simulink library "motion"  (Simulink 4.00)
undefined symbols (not defined in the file or in its folder): A6, Ac, Acd, ad, Aff, Aff0, Aff6, Ap, As, B6, Bc, Bcd, Bff, Bff0, Bff6, Bp, Bs, C6, Cc, Ccd, Cff, Cff0, Cff6, Cp, Cs, D6, Dc, dd, Ddd, Dff, Dff0, Dff6, Dp, Ds, jd, Ts, Tsettle
libraries: motion x5
(part 1 of 4)
settings Model: LastModifiedBy=plambrec

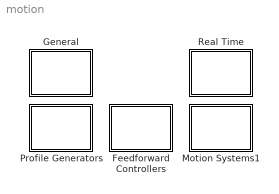
== system motion ==
  Feedforward Controllers : Subsystem
      settings: RTWFcnNameOpts=Auto  RTWFileNameOpts=Auto
      mask Display: disp('Feedforward\nControllers')
  General : Subsystem
      settings: RTWFcnNameOpts=Auto  RTWFileNameOpts=Auto
      mask Display: disp('General')
  Motion Systems1 : Subsystem
      settings: RTWFcnNameOpts=Auto  RTWFileNameOpts=Auto
      mask Display: disp('Motion\nSystems')
  Profile Generators : Subsystem
      settings: RTWFcnNameOpts=Auto  RTWFileNameOpts=Auto
      mask Display: disp('Profile\nGenerators')
  Real Time : Subsystem
      settings: RTWFcnNameOpts=Auto  RTWFileNameOpts=Auto
      mask Display: disp('Real\nTime')

== system motion/Feedforward Controllers ==
  note: Drag Template to
      | Simulink Model Window
  2nd order continuous : Subsystem  mask(Continuous Time Feedforward){m1=30, k1=20}
      mask prompts: m1 "Mass [kg]"; k1 "Actuator to ground Damping [Ns/m]"
      mask help: Continuous Time Feedforward to be used with 2nd order profile generator.
      mask init:
      | m2=0;k2=0;c=1;k12=0;
      | q3=(m1+m2)*c+k1*k2+(k1+k2)*k12;
      | q4=(k1+k2)*c;
      settings: RTWFcnNameOpts=Auto  RTWFileNameOpts=Auto
      mask Help:
      | Continuous Time Feedforward to be used with 2nd order profile generator.
      | See make2.m and look under mask.
      mask Display: disp('Cont. FF')
  2nd order discrete : Subsystem  mask(Discrete Time Feedforward){m1=20, k1=10, Ts=Ts}
      mask prompts: m1 "Actuator Mass [kg]"; k1 "Actuator to ground Damping [Ns/m]"; Ts "Sampling time [s]"
      mask help: Discrete Time Feedforward to be used with 2nd order profile generator.
      mask init:
      | m2=0;k2=0;c=1;k12=0;
      | q2=0;
      settings: RTWFcnNameOpts=Auto  RTWFileNameOpts=Auto
      mask Help:
      | Discrete Time Feedforward to be used with 2nd order profile generator.
      | See make2.m and look under mask.
      mask Display: disp('Disc. FF')
  3d order continuous : Subsystem  mask(Continuous Time Feedforward){m1=30, k1=20, q2=0}
      mask prompts: m1 "Mass [kg]"; k1 "Actuator to ground Damping [Ns/m]"; q2 "Jerk feedforward term (default 0)"
      mask help: Continuous Time Feedforward to be used with 3d order profile generator.
      mask init:
      | m2=0;k2=0;c=1;k12=0;
      | q3=(m1+m2)*c+k1*k2+(k1+k2)*k12;
      | q4=(k1+k2)*c;
      settings: RTWFcnNameOpts=Auto  RTWFileNameOpts=Auto
      mask Help:
      | Continuous Time Feedforward to be used with 3d order profile generator.
      | See make3.m and profile3.m and look under mask.
      mask Display: disp('Cont. FF')
  3d order discrete : Subsystem  mask(Discrete Time Feedforward){m1=20, k1=10, q2=0, Ts=Ts}
      mask prompts: m1 "Actuator Mass [kg]"; k1 "Actuator to ground Damping [Ns/m]"; q2 "Jerk feedforward term (default 0)"; Ts "Sampling time [s]"
      mask help: Discrete Time Feedforward to be used with 3d order profile generator.
      mask init:
      | m2=0;k2=0;c=1;k12=0;
      settings: RTWFcnNameOpts=Auto  RTWFileNameOpts=Auto
      mask Help:
      | Discrete Time Feedforward to be used with 3d order profile generator.
      | See make3.m and profile3.m and look under mask.
      mask Display: disp('Disc. FF')
  4th order  continuous x1 : Subsystem  mask(Continuous Time Feedforward){m1=20, m2=10, k1=10, k2=10, c=6e5, k12=500}
      mask prompts: m1 "Actuator Mass [kg]"; m2 "Load Mass [kg]"; k1 "Actuator to ground Damping [Ns/m]"; k2 "Load to ground Damping [Ns/m]"; c "Spring Stiffness [N/m]"; k12 "Internal Damping [Ns/m]"
      mask help: Continuous Time Feedforward to be used with 4th order profile generator.
      mask init:
      | q1=m1*m2;
      | q2=(m1+m2)*k12+m1*k2+m2*k1;
      | q3=(m1+m2)*c+k1*k2+(k1+k2)*k12;
      | q4=(k1+k2)*c;
      settings: RTWFcnNameOpts=Auto  RTWFileNameOpts=Auto
      mask Help:
      | Continuous Time Feedforward to be used with 4th order profile generator.
      | See make4.m and profile4.m and look under mask.
      mask Display: disp('Cont. FF')
  4th order  discrete x1 : Subsystem  mask(Discrete Time Feedforward){m1=20, m2=10, k1=10, k2=10, c=6e5, k12=500, Ts=Ts}
      mask prompts: m1 "Actuator Mass [kg]"; m2 "Load Mass [kg]"; k1 "Actuator to ground Damping [Ns/m]"; k2 "Load to ground Damping [Ns/m]"; c "Spring Stiffness [N/m]"; k12 "Internal Damping [Ns/m]"; Ts "Sampling time [s]"
      mask help: Discrete Time Feedforward to be used with 4th order profile generator.
      settings: RTWFcnNameOpts=Auto  RTWFileNameOpts=Auto
      mask Help:
      | Discrete Time Feedforward to be used with 4th order profile generator.
      | See make4.m and profile4.m and look under mask.
      mask Display: disp('Disc. FF')
  4th order continuous : Subsystem  mask(Continuous Time Feedforward){m1=20, m2=10, k1=10, k2=10, c=6e5, k12=500}
      mask prompts: m1 "Actuator Mass [kg]"; m2 "Load Mass [kg]"; k1 "Actuator to ground Damping [Ns/m]"; k2 "Load to ground Damping [Ns/m]"; c "Spring Stiffness [N/m]"; k12 "Internal Damping [Ns/m]"
      mask help: Continuous Time Feedforward to be used with 4th order profile generator.
      mask init:
      | q1=m1*m2;
      | q2=(m1+m2)*k12+m1*k2+m2*k1;
      | q3=(m1+m2)*c+k1*k2+(k1+k2)*k12;
      | q4=(k1+k2)*c;
      settings: RTWFcnNameOpts=Auto  RTWFileNameOpts=Auto
      mask Help:
      | Continuous Time Feedforward to be used with 4th order profile generator.
      | See make4.m and profile4.m and look under mask.
      mask Display: disp('Cont. FF')
  4th order digital : Subsystem  mask(Digital Feedforward){m1=20, m2=10, k1=10, k2=10, c=6e5, k12=500, Ts=Ts, r=10*eps}
      mask prompts: m1 "Actuator Mass [kg]"; m2 "Load Mass [kg]"; k1 "Actuator to ground Damping [Ns/m]"; k2 "Load to ground Damping [Ns/m]"; c "Spring Stiffness [N/m]"; k12 "Internal Damping [Ns/m]"; Ts "Sampling time [s]"; r "Resolution of position [m] (default: 10*eps)"
      mask help: Digital Feedforward to be used with 4th order profile generator.
      settings: RTWFcnNameOpts=Auto  RTWFileNameOpts=Auto
      mask Help:
      | Digital Feedforward to be used with 4th order profile generator.
      | See make4.m and profile4.m and look under mask.
      mask Display: disp('Dig. FF')
  4th order discrete : Subsystem  mask(Discrete Time Feedforward){m1=20, m2=10, k1=10, k2=10, c=6e5, k12=500, Ts=Ts}
      mask prompts: m1 "Actuator Mass [kg]"; m2 "Load Mass [kg]"; k1 "Actuator to ground Damping [Ns/m]"; k2 "Load to ground Damping [Ns/m]"; c "Spring Stiffness [N/m]"; k12 "Internal Damping [Ns/m]"; Ts "Sampling time [s]"
      mask help: Discrete Time Feedforward to be used with 4th order profile generator.
      settings: RTWFcnNameOpts=Auto  RTWFileNameOpts=Auto
      mask Help:
      | Discrete Time Feedforward to be used with 4th order profile generator.
      | See make4.m and profile4.m and look under mask.
      mask Display: disp('Disc. FF')
  Feedforward : Subsystem  BlockChoice=4th order continuous
      settings: TemplateBlock=self  MemberBlocks=2nd order continuous,2nd order discrete,3d order continuous,3d order discrete,4th order continuous,4th order digital,4th order discrete  RTWFcnNameOpts=Auto  RTWFileNameOpts=Auto

== system motion/General ==
  note: used to specify parameters
      | for blocks below
  2nd order plant : StateSpace  A=As  B=Bs  C=Cs  D=Ds  X0=0  Realization=auto  AbsoluteTolerance=auto
  4th order Digital Feedforward : Subsystem  mask(4th Order Digital Feedforward ){t0=.3, x=1, v=1, a=5, j=50, d=1000, Ts=1e-3, r=10*eps, s=15, m1=20, m2=10, k1=10, k2=10, c=6e5, k12=500}
      mask prompts: t0 "Starting time:  t0 [s]"; x "Displacement:  x [m]"; v "Bound on velocity:  vmax [m/s]"; a "Bound on acceleration:  amax [m/s2]"; j "Bound on jerk: jmax [m/s3]"; d "Bound on derivative of jerk:  dmax [m/s4]"; Ts "Sampling time (0 for continuous):  Ts [s]"; r "Resolution of position [m] (default: 10*eps)"; s "Number of decimals for digitized d (default: 15)"; m1 "Actuator Mass [kg]"; m2 "Load Mass [kg]"; k1 "Actuator to ground Damping [Ns/m]"; k2 "Load to ground Damping [Ns/m]"; c "Spring Stiffness [N/m]"; k12 "Internal Damping [Ns/m]"
      mask help: Implements a 4th order trajectory planner and feedforward calculation.
      mask init:
      | if length(r)==0 | length(s)==0
      | 	r=10*eps;
      | 	s=15;
      | end
      | [t,dd]=make4(abs(x),v,a,j,d,Ts,r,s);
      | t01=t0-10*eps;
      | if Ts==0
      |    [dj1,tx1,d1,j1,a1,v1,p1,tt1]=profile4(t,dd(1),.001,0);
      | else
      |    [dj1,tx1,d1,j1,a1,v1,p1,tt1]=profile4(t,dd(1),Ts/10,0);
      | end
      settings: RTWFcnNameOpts=Auto  RTWFileNameOpts=Auto
      mask Help: Look under mask
      mask Display:
      | plot([0 dj1(1,:)+t0],[0 dj1(2,:)])
      | text(0.9*(max(dj1(1,:))+t0),0,'F\nx')
  4th order plant : StateSpace  A=Ap  B=Bp  C=Cp  D=Dp  X0=0  Realization=auto  AbsoluteTolerance=auto
  6th order plant : StateSpace  A=A6  B=B6  C=C6  D=D6  X0=0  Realization=auto  AbsoluteTolerance=auto
  Controller : StateSpace  A=Ac  B=Bc  C=Cc  D=Dc  X0=0  Realization=auto  AbsoluteTolerance=auto
  Discrete controller : DiscreteStateSpace  A=Acd  B=Bcd*1.4  C=Ccd  D=Ddd  X0=0  SampleTime=Ts  Realization=auto
  FF: 4th order k12=0 : StateSpace  A=Aff0  B=Bff0  C=Cff0  D=Dff0  X0=0  Realization=auto  AbsoluteTolerance=auto
  FF: 6th order tuning : StateSpace  A=Aff6  B=Bff6  C=Cff6  D=Dff6  X0=0  Realization=auto  AbsoluteTolerance=auto
  FF: Ideal 4th order : StateSpace  A=Aff  B=Bff  C=Cff  D=Dff  X0=0  Realization=auto  AbsoluteTolerance=auto
  open example : Subsystem
      settings: OpenFcn=motion_example1  RTWFcnNameOpts=Auto  RTWFileNameOpts=Auto
      mask Type: Model Opener
      mask Description: Opens Simulink model
      mask Display: disp('EXAMPLE 1\ndoubleclick to open')
  open example1 : Subsystem
      settings: RTWFcnNameOpts=Auto  RTWFileNameOpts=Auto
      settings: OpenFcn=|
      | makeplant
      | motion_example3
      mask Type: Model Opener
      mask Description: Opens Simulink model
      mask Display: disp('EXAMPLE 3\ndoubleclick to open')
  open example2 : Subsystem
      settings: RTWFcnNameOpts=Auto  RTWFileNameOpts=Auto
      settings: OpenFcn=|
      | makeplant
      | motion_example2
      mask Type: Model Opener
      mask Description: Opens Simulink model
      mask Display: disp('EXAMPLE 2\ndoubleclick to open')
  run makeplant : Subsystem
      settings: OpenFcn=makeplant  MoveFcn=edit makeplant  RTWFcnNameOpts=Auto  RTWFileNameOpts=Auto
      mask Type: Script Runner
      mask Description: Run Matlab .M script
      mask Help:
      | This is a convenient block to edit and run a Matlab .M scriptfile from the Simulink environment.
      | Typically such a script is used to define simulation and system parameters.
      | 
      | As an example the scriptfile MAKEPLANT.m is supplied: you may edit this file or use your own.
      | 
      | Double clicking this block will run the script, moving it will start the Matlab editor.
      | 
      | A different script file name can be specified by editing the Callback functions OpenFcn and MoveFcn
      | (see Block Properties)
      mask Display: disp('MAKEPLANT\ndoubleclick to run\nmove to edit')

== system motion/Motion Systems1 ==
  note: Drag Template to
      | Simulink Model Window
  2nd order : StateSpace  A=As  B=Bs  C=Cs  D=Ds  X0=0  Realization=auto  AbsoluteTolerance=auto
  4th order : StateSpace  A=Ap  B=Bp  C=Cp  D=Dp  X0=0  Realization=auto  AbsoluteTolerance=auto
  6th order : StateSpace  A=A6  B=B6  C=C6  D=D6  X0=0  Realization=auto  AbsoluteTolerance=auto
  Motion System : Subsystem  BlockChoice=2nd order
      settings: TemplateBlock=self  MemberBlocks=2nd order,4th order,6th order,Parametrized 4th order  RTWFcnNameOpts=Auto  RTWFileNameOpts=Auto
  Parametrized 4th order : Subsystem  mask(Parametrized 4th order motion system model){m1=20, m2=10, k1=100, k2=100, c=6e5, k12=500}
      mask prompts: m1 "Actuator Mass [kg]"; m2 "Load Mass [kg]"; k1 "Actuator to ground Damping [Ns/m]"; k2 "Load to ground Damping [Ns/m]"; c "Spring Stiffness [N/m]"; k12 "Internal Damping [Ns/m]"
      mask help: Parametrized 4th order motion system model
      mask init:
      | Ap = [   0         1         0         0             % x1
      |        -c/m1  -(k1+k12)/m1  c/m1     k12/m1          % x1dot
      |          0         0         0         1             % x2
      |         c/m2     k12/m2    -c/m2  -(k2+k12)/m2 ];    % x2dot
      | Bp = [   0
      |         1/m1     
      |          0
      |          0   ];
      | Cp = [   0         0        1         0     ];      % x2
      | Dp=0;
      settings: RTWFcnNameOpts=Auto  RTWFileNameOpts=Auto
      mask Help: Parametrized 4th order motion system model
      mask Display: disp('4th order')

== system motion/Profile Generators ==
  note: Drag Template to
      | Simulink Model Window
  Acceleration : Subsystem  mask(2nd Order Profile Generator){t0=.3, x=1, v=1, a=5, Ts=0}
      mask prompts: t0 "Starting time:  t0 [s]"; x "Displacement:  x [m]"; v "Bound on velocity:  vmax [m/s]"; a "Bound on acceleration:  amax [m/s2]"; Ts "Sampling time (0 for continuous):  Ts [s]"
      mask help: 2nd Order Profile Generator
      mask init:
      | [t,ad,aa,tx,a,v,p,tt] = make2(abs(x),v,a,Ts,0);
      | t0=t0-10*eps;
      settings: RTWFcnNameOpts=Auto  RTWFileNameOpts=Auto
      mask Help: See make2.m and look under mask
      mask Display:
      | plot([0 aa(1,:)+t0],[0 aa(2,:)])
      | text(0.8*(max(aa(1,:))+t0),0,'a\n')
  Derivative of Jerk : Subsystem  AncestorBlock=library/Derivative of jerk profile generator  mask(4th Order Profile Generator){t0=.3, x=1, v=1, a=5, j=50, d=1000, Ts=0}
      mask prompts: t0 "Starting time:  t0 [s]"; x "Displacement:  x [m]"; v "Bound on velocity:  vmax [m/s]"; a "Bound on acceleration:  amax [m/s2]"; j "Bound on jerk: jmax [m/s3]"; d "Bound on derivative of jerk:  dmax [m/s4]"; Ts "Sampling time (0 for continuous):  Ts [s]"
      mask help: 4th Order Profile Generator
      mask init:
      | [t,dd]=make4(abs(x),v,a,j,d,Ts);
      | t0=t0-10*eps;
      | [dj,tx,d,j,a,v,p,tt]=profile4(t,dd(1),0,0);
      settings: RTWFcnNameOpts=Auto  RTWFileNameOpts=Auto
      mask Help: See make4.m and profile4.m and look under mask
      mask Display:
      | plot([0 dj(1,:)+t0],[0 dj(2,:)])
      | text(0.8*(max(dj(1,:))+t0),0,'d\n')
  Jerk : Subsystem  mask(3d Order Profile Generator){t0=.3, x=1, v=1, a=5, j=50, Ts=0}
      mask prompts: t0 "Starting time:  t0 [s]"; x "Displacement:  x [m]"; v "Bound on velocity:  vmax [m/s]"; a "Bound on acceleration:  amax [m/s2]"; j "Bound on jerk: jmax [m/s3]"; Ts "Sampling time (0 for continuous):  Ts [s]"
      mask help: 3d Order Profile Generator
      mask init:
      | [t,jd]=make3(abs(x),v,a,j,Ts);
      | t0=t0-10*eps;
      | [jj,tx,j,a,v,p,tt]=profile3(t,jd(1),0,0);
      settings: RTWFcnNameOpts=Auto  RTWFileNameOpts=Auto
      mask Help: See make3.m and profile3.m and look under mask
      mask Display:
      | plot([0 jj(1,:)+t0],[0 jj(2,:)])
      | text(0.85*(max(jj(1,:))+t0),0,'j\n')
  Profile Generator : Subsystem  BlockChoice=Acceleration
      settings: TemplateBlock=self  MemberBlocks=Acceleration,Derivative of Jerk,Jerk,dJerk with error correction  RTWFcnNameOpts=Auto  RTWFileNameOpts=Auto
  dJerk with error correction : Subsystem  mask(4th Order Profile Generator with quantization error correction){t0=.3, x=1, v=1, a=5, j=50, d=1000, Ts=0, r=10*eps, s=15}
      mask prompts: t0 "Starting time:  t0 [s]"; x "Displacement:  x [m]"; v "Bound on velocity:  vmax [m/s]"; a "Bound on acceleration:  amax [m/s2]"; j "Bound on jerk: jmax [m/s3]"; d "Bound on derivative of jerk:  dmax [m/s4]"; Ts "Sampling time (0 for continuous):  Ts [s]"; r "Resolution of position [m] (default: 10*eps)"; s "Number of decimals for digitized d (default: 15)"
      mask help: 4th Order Profile Generator with quantization error correction
      mask init:
      | if length(r)==0 | length(s)==0
      | 	r=10*eps;
      | 	s=15;
      | end
      | [t,dd]=make4(abs(x),v,a,j,d,Ts,r,s);
      | t0=t0-10*eps;
      | [dj,tx,d,j,a,v,p,tt]=profile4(t,dd(1),0,0);
      settings: RTWFcnNameOpts=Auto  RTWFileNameOpts=Auto
      mask Help: See make4.m and profile4.m and look under mask
      mask Display:
      | plot([0 dj(1,:)+t0],[0 dj(2,:)])
      | text(0.8*(max(dj(1,:))+t0),0,'d\n')

== system motion/Real Time ==
  1 : Constant  Value=1
  2 : Constant  Value=0
  Demux : Demux  Outputs=[1 1 5]  BusSelectionMode=off
  Demux1 : Demux  Outputs=[1 1 5]  BusSelectionMode=off
  Generate Feedforward : Subsystem  mask{m1=20, m2=10, k1=10, k2=10, c=6e5, k12=500, Ts=Ts, S1=1, S2=1}
      mask prompts: m1 "Actuator Mass [kg]"; m2 "Load Mass [kg]"; k1 "Actuator Damping [Ns/m]"; k2 "Load Damping [Ns/m]"; c "Stiffness [N/m]"; k12 "Internal Damping [Ns/m]"; Ts "Sample Time [s]"; S1 "Select: 4th order(1) or rigid body(0)"; S2 "Select: actuator(1) or load(0) pos mmnt"
      settings: RTWFcnNameOpts=Auto  RTWFileNameOpts=Auto
  Generate Feedforward with reset : Subsystem  mask{m1=20, m2=10, k1=10, k2=10, c=6e5, k12=500, Ts=Ts, S1=1, S2=1}
      mask prompts: m1 "Actuator Mass [kg]"; m2 "Load Mass [kg]"; k1 "Actuator Damping [Ns/m]"; k2 "Load Damping [Ns/m]"; c "Stiffness [N/m]"; k12 "Internal Damping [Ns/m]"; Ts "Sample Time [s]"; S1 "Select: 4th order(1) or rigid body(0)"; S2 "Select: actuator(1) or load(0) pos mmnt"
      settings: RTWFcnNameOpts=Auto  RTWFileNameOpts=Auto
  Generate Profile : Subsystem  mask{Ts=Ts, Tset=Tsettle, Sdir=1}
      mask prompts: Ts "Sample time [s]"; Tset "Settling time [s]"; Sdir "Switch direction when enabled: 1/0"
      settings: RTWFcnNameOpts=Auto  RTWFileNameOpts=Auto
  Generate Profile with reset : Subsystem  mask{Ts=Ts, Tset=Tsettle, Sdir=1}
      mask prompts: Ts "Sample time [s]"; Tset "Settling time [s]"; Sdir "Switch direction when enabled: 1/0"
      settings: RTWFcnNameOpts=Auto  RTWFileNameOpts=Auto
  Memory1 : Memory  X0=0  InheritSampleTime=on
  Memory2 : Memory  X0=0  InheritSampleTime=on
  Plan Trajectory : Subsystem  TreatAsAtomicUnit=on
      settings: RTWFcnNameOpts=Auto  RTWFileNameOpts=Auto
  Plan Trajectory (with displays) : Subsystem  TreatAsAtomicUnit=on
      settings: RTWFcnNameOpts=Auto  RTWFileNameOpts=Auto
  Terminator1 : Terminator
  Terminator7 : Terminator
  "X-Y planner " : Subsystem  mask{Ts=1/4000, Tsettle=1, X=[ 0 0 ; 0.2 0.2 ; 0.2 -0.2 ; -0.2 -0.2 ; -0.2 0.2 ]}
      mask prompts: Ts "Sampling time [s]"; Tsettle "Settling time (after each move) [s]"; X "Waypoints [ [x1 y1] ; [x2 y2] ; .....]"
      settings: RTWFcnNameOpts=Auto  RTWFileNameOpts=Auto
  open example : Subsystem
      settings: OpenFcn=ref4_rt  RTWFcnNameOpts=Auto  RTWFileNameOpts=Auto
      mask Type: Model Opener
      mask Description: Opens Simulink model
      mask Display: disp('EXAMPLE\ndoubleclick to open')
  open example1 : Subsystem
      settings: OpenFcn=ref4_xy  RTWFcnNameOpts=Auto  RTWFileNameOpts=Auto
      mask Type: Model Opener
      mask Description: Opens Simulink model
      mask Display: disp('EXAMPLE\ndoubleclick to open')
  wires:
  Generate Profile/1(djerk) -> Generate Feedforward/1(djerk)
  Generate Profile with reset/2(reset) -> Generate Feedforward with reset/2(reset)
  Generate Profile with reset/1(djerk) -> Generate Feedforward with reset/1(djerk)
  Generate Profile/2(start) -> Plan Trajectory/Trigger
  Memory2/1 -> Generate Profile/1(t,d)
  Plan Trajectory/1(t,d) -> Memory2/1
  Generate Profile with reset/3(start) -> Plan Trajectory (with displays)/Trigger
  Memory1/1 -> Generate Profile with reset/1(t,d)
  Plan Trajectory (with displays)/1(t,d) -> Memory1/1
  Demux/2 -> [Xref]
  Demux/3 -> Terminator7/1
  Demux/1 -> [FffX]
  "X-Y planner "/1(X) -> Demux/1
  Demux1/2 -> [Yref]
  Demux1/3 -> Terminator1/1
  Demux1/1 -> [FffY]
  "X-Y planner "/2(Y) -> Demux1/1
  1/1 -> "X-Y planner "/1("Cont ")
  2/1 -> "X-Y planner "/2(Trig)

== system motion/Feedforward Controllers/2nd order continuous ==
  note: Rigid Body Feedforward
  note: a
  In1 : Inport  Port=1
  Constant : Constant  Value=0
  Constant1 : Constant  Value=0
  Mux : Mux  Inputs=7
  Position : Integrator  ExternalReset=none  InitialConditionSource=internal  InitialCondition=0  LimitOutput=off  UpperSaturationLimit=inf  LowerSaturationLimit=-inf  ShowSaturationPort=off  ShowStatePort=off  AbsoluteTolerance=auto
  Sum2 : Sum  Orientation=down  Inputs=++|  SaturateOnIntegerOverflow=on
  Velocity : Integrator  ExternalReset=none  InitialConditionSource=internal  InitialCondition=0  LimitOutput=off  UpperSaturationLimit=inf  LowerSaturationLimit=-inf  ShowSaturationPort=off  ShowStatePort=off  AbsoluteTolerance=auto
  filter : TransferFcn  Orientation=down  Numerator=[1]  Denominator=[c]  Realization=auto  AbsoluteTolerance=auto
  m : Gain  Gain=q3  Multiplication=Element-wise(K.*u)  SaturateOnIntegerOverflow=on
  m1 : Gain  Gain=q4  Multiplication=Element-wise(K.*u)  SaturateOnIntegerOverflow=on
  rigid body : Subsystem
      settings: RTWFcnNameOpts=Auto  RTWFileNameOpts=Auto
      mask Display: disp('')
  Out1 : Outport  Port=1
  wires:
  Mux/1 -> Out1/1
  filter/1 -> Mux/1  "feedforward force"
  m/1 -> Sum2/2
  m1/1 -> Sum2/1
  Sum2/1 -> filter/1
  Position/1 -> Mux/2, [p]  "reference"
  Velocity/1 -> Position/1, m1/1, [v]
  In1/1 -> Velocity/1, m/1, [a]
  [p] -> Mux/7  "position"
  Constant/1 -> Mux/3  "derivative of jerk"
  Constant1/1 -> Mux/4  "jerk"
  [a] -> Mux/5  "acceleration"
  [v] -> Mux/6  "velocity"

== system motion/Feedforward Controllers/2nd order discrete ==
  In1 : Inport  Port=1
  (k1+k2)*c : Gain  Gain=(k1+k2)*c  Multiplication=Element-wise(K.*u)  SaturateOnIntegerOverflow=on
  (m1+m2)*c+k1*k2+(k1+k2)*k12 : Gain  Gain=(m1+m2)*c+k1*k2+(k1+k2)*k12  Multiplication=Element-wise(K.*u)  SaturateOnIntegerOverflow=on
  1/c : Gain  Gain=1/c  Multiplication=Element-wise(K.*u)  SaturateOnIntegerOverflow=on
  Constant{,1..3} (4 alike) : Constant  Value=0
  Discrete variable delay : Subsystem  mask{Ts=Ts, alpha=.5}
      mask prompts: Ts "Sample time"; alpha "Delay factor (between 0 and 1)"
      settings: RTWFcnNameOpts=Auto  RTWFileNameOpts=Auto
      mask Display: disp(sprintf('%3.1f*Ts',alpha))
  Discrete variable delay1 : Subsystem  mask{Ts=Ts, alpha=.5}
      mask prompts: Ts "Sample time"; alpha "Delay factor (between 0 and 1)"
      settings: RTWFcnNameOpts=Auto  RTWFileNameOpts=Auto
      mask Display: disp(sprintf('%3.1f*Ts',alpha))
  Discrete variable delay2 : Subsystem  mask{Ts=Ts, alpha=.5}
      mask prompts: Ts "Sample time"; alpha "Delay factor (between 0 and 1)"
      settings: RTWFcnNameOpts=Auto  RTWFileNameOpts=Auto
      mask Display: disp(sprintf('%3.1f*Ts',alpha))
  Mux1 : Mux  Inputs=3
  Mux2 : Mux  Inputs=5
  Sum1 : Sum  Inputs=++++  SaturateOnIntegerOverflow=on
  Unit Delay{1..3,5} (4 alike) : UnitDelay  X0=0  SampleTime=Ts
  ZOH1 : ZeroOrderHold  SampleTime=Ts
  m1*m2 : Gain  Gain=m1*m2  Multiplication=Element-wise(K.*u)  SaturateOnIntegerOverflow=on
  position : DiscreteIntegrator  IntegratorMethod=ForwardEuler  ExternalReset=none  InitialConditionSource=internal  InitialCondition=0  LimitOutput=off  UpperSaturationLimit=inf  LowerSaturationLimit=-inf  ShowSaturationPort=off  ShowStatePort=off  SampleTime=Ts
  q2 : Gain  Gain=q2  Multiplication=Element-wise(K.*u)  SaturateOnIntegerOverflow=on
  velocity : DiscreteIntegrator  IntegratorMethod=ForwardEuler  ExternalReset=none  InitialConditionSource=internal  InitialCondition=0  LimitOutput=off  UpperSaturationLimit=inf  LowerSaturationLimit=-inf  ShowSaturationPort=off  ShowStatePort=off  SampleTime=Ts
  Out1 : Outport  Port=1
  wires:
  [mon] -> Mux1/3
  [ref] -> Mux1/2
  [force] -> Mux1/1
  Mux1/1 -> Out1/1
  Mux2/1 -> [mon]
  velocity/1 -> position/1, [v]
  ZOH1/1 -> velocity/1, [a]  "derivative of jerk"
  position/1 -> [p]
  [p] -> Mux2/5  "position"
  Constant/1 -> Mux2/1  "derivative of jerk"
  Constant3/1 -> Mux2/2  "jerk"
  [a] -> Mux2/3  "acceleration"
  [v] -> Mux2/4  "velocity"
  Constant1/1 -> Unit Delay5/1
  Constant2/1 -> Unit Delay2/1
  [a] -> Unit Delay3/1
  [v] -> Discrete variable delay1/1(In1)
  (m1+m2)*c+k1*k2+(k1+k2)*k12/1 -> Sum1/3
  (k1+k2)*c/1 -> Sum1/4
  Sum1/1 -> 1/c/1
  [p] -> Discrete variable delay/1(In1)
  Discrete variable delay/1(Out1) -> [ref]
  Unit Delay5/1 -> Unit Delay1/1
  Unit Delay1/1 -> m1*m2/1
  Unit Delay2/1 -> Discrete variable delay2/1(In1)
  Unit Delay3/1 -> (m1+m2)*c+k1*k2+(k1+k2)*k12/1
  Discrete variable delay1/1(Out1) -> (k1+k2)*c/1
  Discrete variable delay2/1(Out1) -> q2/1
  1/c/1 -> [force]
  q2/1 -> Sum1/2
  m1*m2/1 -> Sum1/1
  In1/1 -> ZOH1/1

== system motion/Feedforward Controllers/3d order continuous ==
  note: j
  note: Rigid Body Feedforward
  In1 : Inport  Port=1
  Acceleration : Integrator  ExternalReset=none  InitialConditionSource=internal  InitialCondition=0  LimitOutput=off  UpperSaturationLimit=inf  LowerSaturationLimit=-inf  ShowSaturationPort=off  ShowStatePort=off  AbsoluteTolerance=auto
  Constant : Constant  Value=0
  Mux : Mux  Inputs=7
  Position : Integrator  ExternalReset=none  InitialConditionSource=internal  InitialCondition=0  LimitOutput=off  UpperSaturationLimit=inf  LowerSaturationLimit=-inf  ShowSaturationPort=off  ShowStatePort=off  AbsoluteTolerance=auto
  Sum2 : Sum  Orientation=down  Inputs=++|  SaturateOnIntegerOverflow=on
  Sum5 : Sum  Orientation=down  Inputs=++|  SaturateOnIntegerOverflow=on
  Velocity : Integrator  ExternalReset=none  InitialConditionSource=internal  InitialCondition=0  LimitOutput=off  UpperSaturationLimit=inf  LowerSaturationLimit=-inf  ShowSaturationPort=off  ShowStatePort=off  AbsoluteTolerance=auto
  filter : TransferFcn  Orientation=down  Numerator=[1]  Denominator=[c]  Realization=auto  AbsoluteTolerance=auto
  m : Gain  Gain=q3  Multiplication=Element-wise(K.*u)  SaturateOnIntegerOverflow=on
  m1 : Gain  Gain=q4  Multiplication=Element-wise(K.*u)  SaturateOnIntegerOverflow=on
  m2 : Gain  Gain=q2  Multiplication=Element-wise(K.*u)  SaturateOnIntegerOverflow=on
  rigid body : Subsystem
      settings: RTWFcnNameOpts=Auto  RTWFileNameOpts=Auto
      mask Display: disp('')
  Out1 : Outport  Port=1
  wires:
  [v] -> Mux/6  "velocity"
  [a] -> Mux/5  "acceleration"
  [j] -> Mux/4  "jerk"
  Constant/1 -> Mux/3  "derivative of jerk"
  [p] -> Mux/7  "position"
  In1/1 -> [j], m2/1, Acceleration/1
  Velocity/1 -> [v], m1/1, Position/1
  Position/1 -> [p], Mux/2  "reference"
  Sum2/1 -> filter/1
  m1/1 -> Sum2/1
  Acceleration/1 -> [a], m/1, Velocity/1
  m/1 -> Sum5/1
  Sum5/1 -> Sum2/2
  m2/1 -> Sum5/2
  filter/1 -> Mux/1  "feedforward force"
  Mux/1 -> Out1/1

== system motion/Feedforward Controllers/3d order discrete ==
  In1 : Inport  Port=1
  (k1+k2)*c : Gain  Gain=(k1+k2)*c  Multiplication=Element-wise(K.*u)  SaturateOnIntegerOverflow=on
  (m1+m2)*c+k1*k2+(k1+k2)*k12 : Gain  Gain=(m1+m2)*c+k1*k2+(k1+k2)*k12  Multiplication=Element-wise(K.*u)  SaturateOnIntegerOverflow=on
  1/c : Gain  Gain=1/c  Multiplication=Element-wise(K.*u)  SaturateOnIntegerOverflow=on
  Constant : Constant  Value=0
  Constant1 : Constant  Value=0
  Discrete variable delay : Subsystem  mask{Ts=Ts, alpha=.5}
      mask prompts: Ts "Sample time"; alpha "Delay factor (between 0 and 1)"
      settings: RTWFcnNameOpts=Auto  RTWFileNameOpts=Auto
      mask Display: disp(sprintf('%3.1f*Ts',alpha))
  Discrete variable delay1 : Subsystem  mask{Ts=Ts, alpha=.5}
      mask prompts: Ts "Sample time"; alpha "Delay factor (between 0 and 1)"
      settings: RTWFcnNameOpts=Auto  RTWFileNameOpts=Auto
      mask Display: disp(sprintf('%3.1f*Ts',alpha))
  Discrete variable delay2 : Subsystem  mask{Ts=Ts, alpha=.5}
      mask prompts: Ts "Sample time"; alpha "Delay factor (between 0 and 1)"
      settings: RTWFcnNameOpts=Auto  RTWFileNameOpts=Auto
      mask Display: disp(sprintf('%3.1f*Ts',alpha))
  Mux1 : Mux  Inputs=3
  Mux2 : Mux  Inputs=5
  Sum1 : Sum  Inputs=++++  SaturateOnIntegerOverflow=on
  Unit Delay{1..3,5} (4 alike) : UnitDelay  X0=0  SampleTime=Ts
  ZOH1 : ZeroOrderHold  SampleTime=Ts
  acceleration : DiscreteIntegrator  IntegratorMethod=ForwardEuler  ExternalReset=none  InitialConditionSource=internal  InitialCondition=0  LimitOutput=off  UpperSaturationLimit=inf  LowerSaturationLimit=-inf  ShowSaturationPort=off  ShowStatePort=off  SampleTime=Ts
  m1*m2 : Gain  Gain=m1*m2  Multiplication=Element-wise(K.*u)  SaturateOnIntegerOverflow=on
  position : DiscreteIntegrator  IntegratorMethod=ForwardEuler  ExternalReset=none  InitialConditionSource=internal  InitialCondition=0  LimitOutput=off  UpperSaturationLimit=inf  LowerSaturationLimit=-inf  ShowSaturationPort=off  ShowStatePort=off  SampleTime=Ts
  q2 : Gain  Gain=q2  Multiplication=Element-wise(K.*u)  SaturateOnIntegerOverflow=on
  velocity : DiscreteIntegrator  IntegratorMethod=ForwardEuler  ExternalReset=none  InitialConditionSource=internal  InitialCondition=0  LimitOutput=off  UpperSaturationLimit=inf  LowerSaturationLimit=-inf  ShowSaturationPort=off  ShowStatePort=off  SampleTime=Ts
  Out1 : Outport  Port=1
  wires:
  In1/1 -> ZOH1/1
  m1*m2/1 -> Sum1/1
  q2/1 -> Sum1/2
  1/c/1 -> [force]
  Discrete variable delay2/1(Out1) -> q2/1
  Discrete variable delay1/1(Out1) -> (k1+k2)*c/1
  Unit Delay3/1 -> (m1+m2)*c+k1*k2+(k1+k2)*k12/1
  Unit Delay2/1 -> Discrete variable delay2/1(In1)
  Unit Delay1/1 -> m1*m2/1
  Unit Delay5/1 -> Unit Delay1/1
  Discrete variable delay/1(Out1) -> [ref]
  [p] -> Discrete variable delay/1(In1)
  Sum1/1 -> 1/c/1
  (k1+k2)*c/1 -> Sum1/4
  (m1+m2)*c+k1*k2+(k1+k2)*k12/1 -> Sum1/3
  [v] -> Discrete variable delay1/1(In1)
  [a] -> Unit Delay3/1
  [j] -> Unit Delay2/1
  Constant1/1 -> Unit Delay5/1
  [v] -> Mux2/4  "velocity"
  [a] -> Mux2/3  "acceleration"
  [j] -> Mux2/2  "jerk"
  Constant/1 -> Mux2/1  "derivative of jerk"
  [p] -> Mux2/5  "position"
  position/1 -> [p]
  ZOH1/1 -> [j], acceleration/1  "derivative of jerk"
  velocity/1 -> [v], position/1
  acceleration/1 -> [a], velocity/1
  Mux2/1 -> [mon]
  Mux1/1 -> Out1/1
  [force] -> Mux1/1
  [ref] -> Mux1/2
  [mon] -> Mux1/3

== system motion/Feedforward Controllers/4th order  continuous x1 ==
  note: d
  note: Rigid Body Feedforward
  In1 : Inport  Port=1
  Acceleration : Integrator  ExternalReset=none  InitialConditionSource=internal  InitialCondition=0  LimitOutput=off  UpperSaturationLimit=inf  LowerSaturationLimit=-inf  ShowSaturationPort=off  ShowStatePort=off  AbsoluteTolerance=auto
  Jerk : Integrator  ExternalReset=none  InitialConditionSource=internal  InitialCondition=0  LimitOutput=off  UpperSaturationLimit=inf  LowerSaturationLimit=-inf  ShowSaturationPort=off  ShowStatePort=off  AbsoluteTolerance=auto
  Mux : Mux  Inputs=7
  Position : Integrator  ExternalReset=none  InitialConditionSource=internal  InitialCondition=0  LimitOutput=off  UpperSaturationLimit=inf  LowerSaturationLimit=-inf  ShowSaturationPort=off  ShowStatePort=off  AbsoluteTolerance=auto
  Sum1 : Sum  Inputs=+++  SaturateOnIntegerOverflow=on
  Sum2 : Sum  Orientation=down  Inputs=++|  SaturateOnIntegerOverflow=on
  Sum3 : Sum  Orientation=down  Inputs=++|  SaturateOnIntegerOverflow=on
  Sum5 : Sum  Orientation=down  Inputs=++|  SaturateOnIntegerOverflow=on
  Velocity : Integrator  ExternalReset=none  InitialConditionSource=internal  InitialCondition=0  LimitOutput=off  UpperSaturationLimit=inf  LowerSaturationLimit=-inf  ShowSaturationPort=off  ShowStatePort=off  AbsoluteTolerance=auto
  filter : TransferFcn  Orientation=down  Numerator=[1]  Denominator=[ k12 c]  Realization=auto  AbsoluteTolerance=auto
  filter1 : TransferFcn  Numerator=[1]  Denominator=[ k12 c]  Realization=auto  AbsoluteTolerance=auto
  m : Gain  Gain=q3  Multiplication=Element-wise(K.*u)  SaturateOnIntegerOverflow=on
  m1 : Gain  Gain=q4  Multiplication=Element-wise(K.*u)  SaturateOnIntegerOverflow=on
  m2 : Gain  Gain=q2  Multiplication=Element-wise(K.*u)  SaturateOnIntegerOverflow=on
  m3 : Gain  Gain=q1  Multiplication=Element-wise(K.*u)  SaturateOnIntegerOverflow=on
  m4 : Gain  Gain=k2+k12  Multiplication=Element-wise(K.*u)  SaturateOnIntegerOverflow=on
  m5 : Gain  Gain=m2  Multiplication=Element-wise(K.*u)  SaturateOnIntegerOverflow=on
  m6 : Gain  Gain=c  Multiplication=Element-wise(K.*u)  SaturateOnIntegerOverflow=on
  rigid body : Subsystem
      settings: RTWFcnNameOpts=Auto  RTWFileNameOpts=Auto
      mask Display: disp('')
  Out1 : Outport  Port=1
  wires:
  [v] -> Mux/6  "velocity"
  [a] -> Mux/5  "acceleration"
  [j] -> Mux/4  "jerk"
  [d] -> Mux/3  "derivative of jerk"
  [p] -> Mux/7  "position"
  In1/1 -> [d], m3/1, Jerk/1
  Velocity/1 -> [v], m1/1, Position/1, m4/1
  Position/1 -> [p], m6/1  "reference x2"
  Sum2/1 -> filter/1
  m1/1 -> Sum2/1
  Jerk/1 -> [j], m2/1, Acceleration/1
  Acceleration/1 -> [a], m/1, Velocity/1, m5/1
  m/1 -> Sum5/1
  Sum5/1 -> Sum2/2
  m2/1 -> Sum3/1
  Sum3/1 -> Sum5/2
  m3/1 -> Sum3/2
  filter/1 -> Mux/1  "feedforward force"
  Mux/1 -> Out1/1
  m5/1 -> Sum1/1
  m4/1 -> Sum1/2
  m6/1 -> Sum1/3
  Sum1/1 -> filter1/1  "reference x1"
  filter1/1 -> Mux/2  "reference x1"

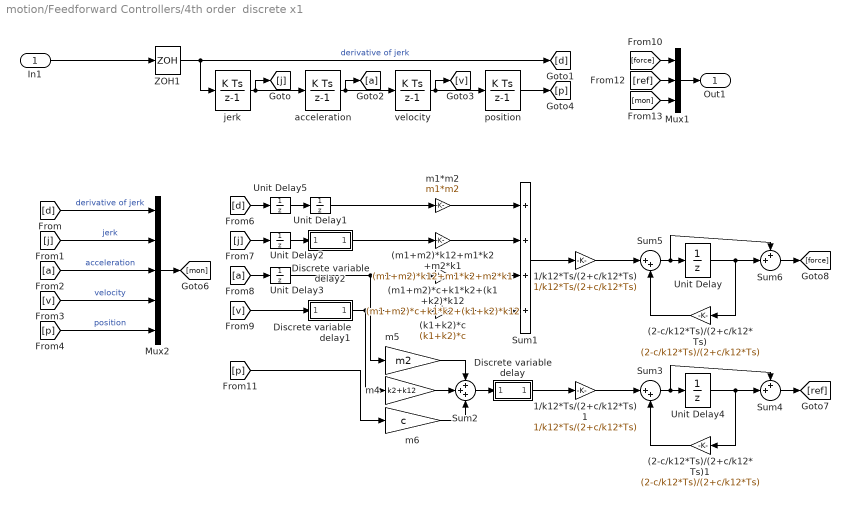
== system motion/Feedforward Controllers/4th order  discrete x1 ==
  In1 : Inport  Port=1
  (2-c/k12*Ts)/(2+c/k12*Ts) : Gain  Orientation=left  Gain=(2-c/k12*Ts)/(2+c/k12*Ts)  Multiplication=Element-wise(K.*u)  SaturateOnIntegerOverflow=on
  (2-c/k12*Ts)/(2+c/k12*Ts)1 : Gain  Orientation=left  Gain=(2-c/k12*Ts)/(2+c/k12*Ts)  Multiplication=Element-wise(K.*u)  SaturateOnIntegerOverflow=on
  (k1+k2)*c : Gain  Gain=(k1+k2)*c  Multiplication=Element-wise(K.*u)  SaturateOnIntegerOverflow=on
  (m1+m2)*c+k1*k2+(k1+k2)*k12 : Gain  Gain=(m1+m2)*c+k1*k2+(k1+k2)*k12  Multiplication=Element-wise(K.*u)  SaturateOnIntegerOverflow=on
  (m1+m2)*k12+m1*k2+m2*k1 : Gain  Gain=(m1+m2)*k12+m1*k2+m2*k1  Multiplication=Element-wise(K.*u)  SaturateOnIntegerOverflow=on
  1/k12*Ts/(2+c/k12*Ts) : Gain  Gain=1/k12*Ts/(2+c/k12*Ts)  Multiplication=Element-wise(K.*u)  SaturateOnIntegerOverflow=on
  1/k12*Ts/(2+c/k12*Ts)1 : Gain  Gain=1/k12*Ts/(2+c/k12*Ts)  Multiplication=Element-wise(K.*u)  SaturateOnIntegerOverflow=on
  Discrete variable delay : Subsystem  mask{Ts=Ts, alpha=.5}
      mask prompts: Ts "Sample time"; alpha "Delay factor (between 0 and 1)"
      settings: RTWFcnNameOpts=Auto  RTWFileNameOpts=Auto
      mask Display: disp(sprintf('%3.1f*Ts',alpha))
  Discrete variable delay1 : Subsystem  mask{Ts=Ts, alpha=.5}
      mask prompts: Ts "Sample time"; alpha "Delay factor (between 0 and 1)"
      settings: RTWFcnNameOpts=Auto  RTWFileNameOpts=Auto
      mask Display: disp(sprintf('%3.1f*Ts',alpha))
  Discrete variable delay2 : Subsystem  mask{Ts=Ts, alpha=.5}
      mask prompts: Ts "Sample time"; alpha "Delay factor (between 0 and 1)"
      settings: RTWFcnNameOpts=Auto  RTWFileNameOpts=Auto
      mask Display: disp(sprintf('%3.1f*Ts',alpha))
  Mux1 : Mux  Inputs=3
  Mux2 : Mux  Inputs=5
  Sum1 : Sum  Inputs=++++  SaturateOnIntegerOverflow=on
  Sum2 : Sum  Inputs=+++  SaturateOnIntegerOverflow=on
  Sum3 : Sum  Inputs=|++  SaturateOnIntegerOverflow=on
  Sum4 : Sum  Inputs=++|  SaturateOnIntegerOverflow=on
  Sum5 : Sum  Inputs=|++  SaturateOnIntegerOverflow=on
  Sum6 : Sum  Inputs=++|  SaturateOnIntegerOverflow=on
  Unit Delay{,1..5} (6 alike) : UnitDelay  X0=0  SampleTime=Ts
  ZOH1 : ZeroOrderHold  SampleTime=Ts
  acceleration : DiscreteIntegrator  IntegratorMethod=ForwardEuler  ExternalReset=none  InitialConditionSource=internal  InitialCondition=0  LimitOutput=off  UpperSaturationLimit=inf  LowerSaturationLimit=-inf  ShowSaturationPort=off  ShowStatePort=off  SampleTime=Ts
  jerk : DiscreteIntegrator  IntegratorMethod=ForwardEuler  ExternalReset=none  InitialConditionSource=internal  InitialCondition=0  LimitOutput=off  UpperSaturationLimit=inf  LowerSaturationLimit=-inf  ShowSaturationPort=off  ShowStatePort=off  SampleTime=Ts
  m1*m2 : Gain  Gain=m1*m2  Multiplication=Element-wise(K.*u)  SaturateOnIntegerOverflow=on
  m4 : Gain  Gain=k2+k12  Multiplication=Element-wise(K.*u)  SaturateOnIntegerOverflow=on
  m5 : Gain  Gain=m2  Multiplication=Element-wise(K.*u)  SaturateOnIntegerOverflow=on
  m6 : Gain  Gain=c  Multiplication=Element-wise(K.*u)  SaturateOnIntegerOverflow=on
  position : DiscreteIntegrator  IntegratorMethod=ForwardEuler  ExternalReset=none  InitialConditionSource=internal  InitialCondition=0  LimitOutput=off  UpperSaturationLimit=inf  LowerSaturationLimit=-inf  ShowSaturationPort=off  ShowStatePort=off  SampleTime=Ts
  velocity : DiscreteIntegrator  IntegratorMethod=ForwardEuler  ExternalReset=none  InitialConditionSource=internal  InitialCondition=0  LimitOutput=off  UpperSaturationLimit=inf  LowerSaturationLimit=-inf  ShowSaturationPort=off  ShowStatePort=off  SampleTime=Ts
  Out1 : Outport  Port=1
  wires:
  In1/1 -> ZOH1/1
  m1*m2/1 -> Sum1/1
  (m1+m2)*k12+m1*k2+m2*k1/1 -> Sum1/2
  (2-c/k12*Ts)/(2+c/k12*Ts)/1 -> Sum5/2
  Unit Delay/1 -> Sum6/2, (2-c/k12*Ts)/(2+c/k12*Ts)/1
  Sum5/1 -> Sum6/1, Unit Delay/1
  1/k12*Ts/(2+c/k12*Ts)/1 -> Sum5/1
  Discrete variable delay2/1(Out1) -> (m1+m2)*k12+m1*k2+m2*k1/1
  Discrete variable delay1/1(Out1) -> (k1+k2)*c/1, m4/1
  Unit Delay3/1 -> (m1+m2)*c+k1*k2+(k1+k2)*k12/1, m5/1
  Unit Delay2/1 -> Discrete variable delay2/1(In1)
  Unit Delay1/1 -> m1*m2/1
  Unit Delay5/1 -> Unit Delay1/1
  Sum1/1 -> 1/k12*Ts/(2+c/k12*Ts)/1
  (k1+k2)*c/1 -> Sum1/4
  (m1+m2)*c+k1*k2+(k1+k2)*k12/1 -> Sum1/3
  [v] -> Discrete variable delay1/1(In1)
  [a] -> Unit Delay3/1
  [j] -> Unit Delay2/1
  [d] -> Unit Delay5/1
  [v] -> Mux2/4  "velocity"
  [a] -> Mux2/3  "acceleration"
  [j] -> Mux2/2  "jerk"
  [d] -> Mux2/1  "derivative of jerk"
  [p] -> Mux2/5  "position"
  position/1 -> [p]
  ZOH1/1 -> jerk/1, [d]  "derivative of jerk"
  velocity/1 -> [v], position/1
  acceleration/1 -> [a], velocity/1
  jerk/1 -> [j], acceleration/1
  Mux2/1 -> [mon]
  Mux1/1 -> Out1/1
  Sum6/1 -> [force]
  [force] -> Mux1/1
  [ref] -> Mux1/2
  [mon] -> Mux1/3
  m5/1 -> Sum2/1
  m4/1 -> Sum2/2
  m6/1 -> Sum2/3
  [p] -> m6/1
  (2-c/k12*Ts)/(2+c/k12*Ts)1/1 -> Sum3/2
  Unit Delay4/1 -> (2-c/k12*Ts)/(2+c/k12*Ts)1/1, Sum4/2
  Sum3/1 -> Unit Delay4/1, Sum4/1
  1/k12*Ts/(2+c/k12*Ts)1/1 -> Sum3/1
  Sum2/1 -> Discrete variable delay/1(In1)
  Sum4/1 -> [ref]
  Discrete variable delay/1(Out1) -> 1/k12*Ts/(2+c/k12*Ts)1/1

== system motion/Feedforward Controllers/4th order continuous ==
  note: Rigid Body Feedforward
  note: d
  In1 : Inport  Port=1
  Acceleration : Integrator  ExternalReset=none  InitialConditionSource=internal  InitialCondition=0  LimitOutput=off  UpperSaturationLimit=inf  LowerSaturationLimit=-inf  ShowSaturationPort=off  ShowStatePort=off  AbsoluteTolerance=auto
  Jerk : Integrator  ExternalReset=none  InitialConditionSource=internal  InitialCondition=0  LimitOutput=off  UpperSaturationLimit=inf  LowerSaturationLimit=-inf  ShowSaturationPort=off  ShowStatePort=off  AbsoluteTolerance=auto
  Mux : Mux  Inputs=7
  Position : Integrator  ExternalReset=none  InitialConditionSource=internal  InitialCondition=0  LimitOutput=off  UpperSaturationLimit=inf  LowerSaturationLimit=-inf  ShowSaturationPort=off  ShowStatePort=off  AbsoluteTolerance=auto
  Sum2 : Sum  Orientation=down  Inputs=++|  SaturateOnIntegerOverflow=on
  Sum3 : Sum  Orientation=down  Inputs=++|  SaturateOnIntegerOverflow=on
  Sum5 : Sum  Orientation=down  Inputs=++|  SaturateOnIntegerOverflow=on
  Velocity : Integrator  ExternalReset=none  InitialConditionSource=internal  InitialCondition=0  LimitOutput=off  UpperSaturationLimit=inf  LowerSaturationLimit=-inf  ShowSaturationPort=off  ShowStatePort=off  AbsoluteTolerance=auto
  filter : TransferFcn  Orientation=down  Numerator=[1]  Denominator=[ k12 c]  Realization=auto  AbsoluteTolerance=auto
  m : Gain  Gain=q3  Multiplication=Element-wise(K.*u)  SaturateOnIntegerOverflow=on
  m1 : Gain  Gain=q4  Multiplication=Element-wise(K.*u)  SaturateOnIntegerOverflow=on
  m2 : Gain  Gain=q2  Multiplication=Element-wise(K.*u)  SaturateOnIntegerOverflow=on
  m3 : Gain  Gain=q1  Multiplication=Element-wise(K.*u)  SaturateOnIntegerOverflow=on
  rigid body : Subsystem
      settings: RTWFcnNameOpts=Auto  RTWFileNameOpts=Auto
      mask Display: disp('')
  Out1 : Outport  Port=1
  wires:
  Mux/1 -> Out1/1
  filter/1 -> Mux/1  "feedforward force"
  m3/1 -> Sum3/2
  Sum3/1 -> Sum5/2
  m2/1 -> Sum3/1
  Sum5/1 -> Sum2/2
  m/1 -> Sum5/1
  Acceleration/1 -> Velocity/1, m/1, [a]
  Jerk/1 -> Acceleration/1, m2/1, [j]
  m1/1 -> Sum2/1
  Sum2/1 -> filter/1
  Position/1 -> Mux/2, [p]  "reference"
  Velocity/1 -> Position/1, m1/1, [v]
  In1/1 -> Jerk/1, m3/1, [d]
  [p] -> Mux/7  "position"
  [d] -> Mux/3  "derivative of jerk"
  [j] -> Mux/4  "jerk"
  [a] -> Mux/5  "acceleration"
  [v] -> Mux/6  "velocity"

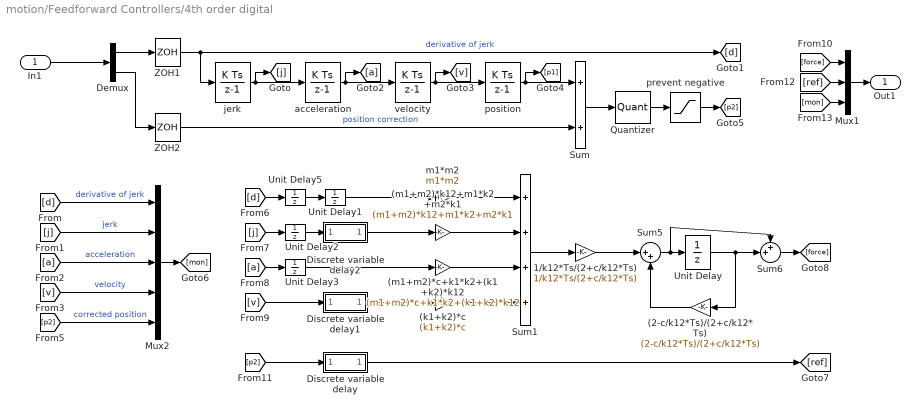
== system motion/Feedforward Controllers/4th order digital ==
  In1 : Inport  Port=1
  (2-c/k12*Ts)/(2+c/k12*Ts) : Gain  Orientation=left  Gain=(2-c/k12*Ts)/(2+c/k12*Ts)  Multiplication=Element-wise(K.*u)  SaturateOnIntegerOverflow=on
  (k1+k2)*c : Gain  Gain=(k1+k2)*c  Multiplication=Element-wise(K.*u)  SaturateOnIntegerOverflow=on
  (m1+m2)*c+k1*k2+(k1+k2)*k12 : Gain  Gain=(m1+m2)*c+k1*k2+(k1+k2)*k12  Multiplication=Element-wise(K.*u)  SaturateOnIntegerOverflow=on
  (m1+m2)*k12+m1*k2+m2*k1 : Gain  Gain=(m1+m2)*k12+m1*k2+m2*k1  Multiplication=Element-wise(K.*u)  SaturateOnIntegerOverflow=on
  1/k12*Ts/(2+c/k12*Ts) : Gain  Gain=1/k12*Ts/(2+c/k12*Ts)  Multiplication=Element-wise(K.*u)  SaturateOnIntegerOverflow=on
  Demux : Demux  Outputs=2  BusSelectionMode=off
  Discrete variable delay : Subsystem  mask{Ts=Ts, alpha=.5}
      mask prompts: Ts "Sample time"; alpha "Delay factor (between 0 and 1)"
      settings: RTWFcnNameOpts=Auto  RTWFileNameOpts=Auto
      mask Display: disp(sprintf('%3.1f*Ts',alpha))
  Discrete variable delay1 : Subsystem  mask{Ts=Ts, alpha=.5}
      mask prompts: Ts "Sample time"; alpha "Delay factor (between 0 and 1)"
      settings: RTWFcnNameOpts=Auto  RTWFileNameOpts=Auto
      mask Display: disp(sprintf('%3.1f*Ts',alpha))
  Discrete variable delay2 : Subsystem  mask{Ts=Ts, alpha=.5}
      mask prompts: Ts "Sample time"; alpha "Delay factor (between 0 and 1)"
      settings: RTWFcnNameOpts=Auto  RTWFileNameOpts=Auto
      mask Display: disp(sprintf('%3.1f*Ts',alpha))
  Mux1 : Mux  Inputs=3
  Mux2 : Mux  Inputs=5
  Quantizer : Quantizer  QuantizationInterval=r  LinearizeAsGain=on
  Sum : Sum  Inputs=++  SaturateOnIntegerOverflow=on
  Sum1 : Sum  Inputs=++++  SaturateOnIntegerOverflow=on
  Sum5 : Sum  Inputs=|++  SaturateOnIntegerOverflow=on
  Sum6 : Sum  Inputs=++|  SaturateOnIntegerOverflow=on
  Unit Delay{,1..3,5} (5 alike) : UnitDelay  X0=0  SampleTime=Ts
  ZOH1 : ZeroOrderHold  SampleTime=Ts
  ZOH2 : ZeroOrderHold  SampleTime=Ts
  acceleration : DiscreteIntegrator  IntegratorMethod=ForwardEuler  ExternalReset=none  InitialConditionSource=internal  InitialCondition=0  LimitOutput=off  UpperSaturationLimit=inf  LowerSaturationLimit=-inf  ShowSaturationPort=off  ShowStatePort=off  SampleTime=Ts
  jerk : DiscreteIntegrator  IntegratorMethod=ForwardEuler  ExternalReset=none  InitialConditionSource=internal  InitialCondition=0  LimitOutput=off  UpperSaturationLimit=inf  LowerSaturationLimit=-inf  ShowSaturationPort=off  ShowStatePort=off  SampleTime=Ts
  m1*m2 : Gain  Gain=m1*m2  Multiplication=Element-wise(K.*u)  SaturateOnIntegerOverflow=on
  position : DiscreteIntegrator  IntegratorMethod=ForwardEuler  ExternalReset=none  InitialConditionSource=internal  InitialCondition=0  LimitOutput=off  UpperSaturationLimit=inf  LowerSaturationLimit=-inf  ShowSaturationPort=off  ShowStatePort=off  SampleTime=Ts
  "prevent negative " : Saturate  UpperLimit=inf  LowerLimit=0  LinearizeAsGain=on
  velocity : DiscreteIntegrator  IntegratorMethod=ForwardEuler  ExternalReset=none  InitialConditionSource=internal  InitialCondition=0  LimitOutput=off  UpperSaturationLimit=inf  LowerSaturationLimit=-inf  ShowSaturationPort=off  ShowStatePort=off  SampleTime=Ts
  Out1 : Outport  Port=1
  wires:
  In1/1 -> Demux/1
  m1*m2/1 -> Sum1/1
  (m1+m2)*k12+m1*k2+m2*k1/1 -> Sum1/2
  (2-c/k12*Ts)/(2+c/k12*Ts)/1 -> Sum5/2
  Unit Delay/1 -> Sum6/2, (2-c/k12*Ts)/(2+c/k12*Ts)/1
  Sum5/1 -> Sum6/1, Unit Delay/1
  1/k12*Ts/(2+c/k12*Ts)/1 -> Sum5/1
  Discrete variable delay2/1(Out1) -> (m1+m2)*k12+m1*k2+m2*k1/1
  Discrete variable delay1/1(Out1) -> (k1+k2)*c/1
  Unit Delay3/1 -> (m1+m2)*c+k1*k2+(k1+k2)*k12/1
  Unit Delay2/1 -> Discrete variable delay2/1(In1)
  Unit Delay1/1 -> m1*m2/1
  Unit Delay5/1 -> Unit Delay1/1
  "prevent negative "/1 -> [p2]
  Discrete variable delay/1(Out1) -> [ref]
  [p2] -> Discrete variable delay/1(In1)
  Sum1/1 -> 1/k12*Ts/(2+c/k12*Ts)/1
  (k1+k2)*c/1 -> Sum1/4
  (m1+m2)*c+k1*k2+(k1+k2)*k12/1 -> Sum1/3
  [v] -> Discrete variable delay1/1(In1)
  [a] -> Unit Delay3/1
  [j] -> Unit Delay2/1
  [d] -> Unit Delay5/1
  [v] -> Mux2/4  "velocity"
  [a] -> Mux2/3  "acceleration"
  [j] -> Mux2/2  "jerk"
  [d] -> Mux2/1  "derivative of jerk"
  [p2] -> Mux2/5  "corrected position"
  ZOH2/1 -> Sum/2  "position correction"
  position/1 -> [p1], Sum/1
  Sum/1 -> Quantizer/1
  Quantizer/1 -> "prevent negative "/1
  Demux/2 -> ZOH2/1
  ZOH1/1 -> jerk/1, [d]  "derivative of jerk"
  velocity/1 -> [v], position/1
  acceleration/1 -> [a], velocity/1
  jerk/1 -> [j], acceleration/1
  Demux/1 -> ZOH1/1
  Mux2/1 -> [mon]
  Mux1/1 -> Out1/1
  Sum6/1 -> [force]
  [force] -> Mux1/1
  [ref] -> Mux1/2
  [mon] -> Mux1/3

== system motion/Feedforward Controllers/4th order discrete ==
  In1 : Inport  Port=1
  (2-c/k12*Ts)/(2+c/k12*Ts) : Gain  Orientation=left  Gain=(2-c/k12*Ts)/(2+c/k12*Ts)  Multiplication=Element-wise(K.*u)  SaturateOnIntegerOverflow=on
  (k1+k2)*c : Gain  Gain=(k1+k2)*c  Multiplication=Element-wise(K.*u)  SaturateOnIntegerOverflow=on
  (m1+m2)*c+k1*k2+(k1+k2)*k12 : Gain  Gain=(m1+m2)*c+k1*k2+(k1+k2)*k12  Multiplication=Element-wise(K.*u)  SaturateOnIntegerOverflow=on
  (m1+m2)*k12+m1*k2+m2*k1 : Gain  Gain=(m1+m2)*k12+m1*k2+m2*k1  Multiplication=Element-wise(K.*u)  SaturateOnIntegerOverflow=on
  1/k12*Ts/(2+c/k12*Ts) : Gain  Gain=1/k12*Ts/(2+c/k12*Ts)  Multiplication=Element-wise(K.*u)  SaturateOnIntegerOverflow=on
  Discrete variable delay : Subsystem  mask{Ts=Ts, alpha=.5}
      mask prompts: Ts "Sample time"; alpha "Delay factor (between 0 and 1)"
      settings: RTWFcnNameOpts=Auto  RTWFileNameOpts=Auto
      mask Display: disp(sprintf('%3.1f*Ts',alpha))
  Discrete variable delay1 : Subsystem  mask{Ts=Ts, alpha=.5}
      mask prompts: Ts "Sample time"; alpha "Delay factor (between 0 and 1)"
      settings: RTWFcnNameOpts=Auto  RTWFileNameOpts=Auto
      mask Display: disp(sprintf('%3.1f*Ts',alpha))
  Discrete variable delay2 : Subsystem  mask{Ts=Ts, alpha=.5}
      mask prompts: Ts "Sample time"; alpha "Delay factor (between 0 and 1)"
      settings: RTWFcnNameOpts=Auto  RTWFileNameOpts=Auto
      mask Display: disp(sprintf('%3.1f*Ts',alpha))
  Mux1 : Mux  Inputs=3
  Mux2 : Mux  Inputs=5
  Sum1 : Sum  Inputs=++++  SaturateOnIntegerOverflow=on
  Sum5 : Sum  Inputs=|++  SaturateOnIntegerOverflow=on
  Sum6 : Sum  Inputs=++|  SaturateOnIntegerOverflow=on
  Unit Delay{,1..3,5} (5 alike) : UnitDelay  X0=0  SampleTime=Ts
  ZOH1 : ZeroOrderHold  SampleTime=Ts
  acceleration : DiscreteIntegrator  IntegratorMethod=ForwardEuler  ExternalReset=none  InitialConditionSource=internal  InitialCondition=0  LimitOutput=off  UpperSaturationLimit=inf  LowerSaturationLimit=-inf  ShowSaturationPort=off  ShowStatePort=off  SampleTime=Ts
  jerk : DiscreteIntegrator  IntegratorMethod=ForwardEuler  ExternalReset=none  InitialConditionSource=internal  InitialCondition=0  LimitOutput=off  UpperSaturationLimit=inf  LowerSaturationLimit=-inf  ShowSaturationPort=off  ShowStatePort=off  SampleTime=Ts
  m1*m2 : Gain  Gain=m1*m2  Multiplication=Element-wise(K.*u)  SaturateOnIntegerOverflow=on
  position : DiscreteIntegrator  IntegratorMethod=ForwardEuler  ExternalReset=none  InitialConditionSource=internal  InitialCondition=0  LimitOutput=off  UpperSaturationLimit=inf  LowerSaturationLimit=-inf  ShowSaturationPort=off  ShowStatePort=off  SampleTime=Ts
  velocity : DiscreteIntegrator  IntegratorMethod=ForwardEuler  ExternalReset=none  InitialConditionSource=internal  InitialCondition=0  LimitOutput=off  UpperSaturationLimit=inf  LowerSaturationLimit=-inf  ShowSaturationPort=off  ShowStatePort=off  SampleTime=Ts
  Out1 : Outport  Port=1
  wires:
  [mon] -> Mux1/3
  [ref] -> Mux1/2
  [force] -> Mux1/1
  Sum6/1 -> [force]
  Mux1/1 -> Out1/1
  Mux2/1 -> [mon]
  jerk/1 -> acceleration/1, [j]
  acceleration/1 -> velocity/1, [a]
  velocity/1 -> position/1, [v]
  ZOH1/1 -> [d], jerk/1  "derivative of jerk"
  position/1 -> [p]
  [p] -> Mux2/5  "position"
  [d] -> Mux2/1  "derivative of jerk"
  [j] -> Mux2/2  "jerk"
  [a] -> Mux2/3  "acceleration"
  [v] -> Mux2/4  "velocity"
  [d] -> Unit Delay5/1
  [j] -> Unit Delay2/1
  [a] -> Unit Delay3/1
  [v] -> Discrete variable delay1/1(In1)
  (m1+m2)*c+k1*k2+(k1+k2)*k12/1 -> Sum1/3
  (k1+k2)*c/1 -> Sum1/4
  Sum1/1 -> 1/k12*Ts/(2+c/k12*Ts)/1
  [p] -> Discrete variable delay/1(In1)
  Discrete variable delay/1(Out1) -> [ref]
  Unit Delay5/1 -> Unit Delay1/1
  Unit Delay1/1 -> m1*m2/1
  Unit Delay2/1 -> Discrete variable delay2/1(In1)
  Unit Delay3/1 -> (m1+m2)*c+k1*k2+(k1+k2)*k12/1
  Discrete variable delay1/1(Out1) -> (k1+k2)*c/1
  Discrete variable delay2/1(Out1) -> (m1+m2)*k12+m1*k2+m2*k1/1
  1/k12*Ts/(2+c/k12*Ts)/1 -> Sum5/1
  Sum5/1 -> Unit Delay/1, Sum6/1
  Unit Delay/1 -> (2-c/k12*Ts)/(2+c/k12*Ts)/1, Sum6/2
  (2-c/k12*Ts)/(2+c/k12*Ts)/1 -> Sum5/2
  (m1+m2)*k12+m1*k2+m2*k1/1 -> Sum1/2
  m1*m2/1 -> Sum1/1
  In1/1 -> ZOH1/1
